simulink model "calc2"  (R2021a)
settings: Solver=VariableStepAuto  StartTime=0.0  StopTime=10.0  RelTol=1e-3
settings Model: Creator=Noha  LastModifiedBy=Noha

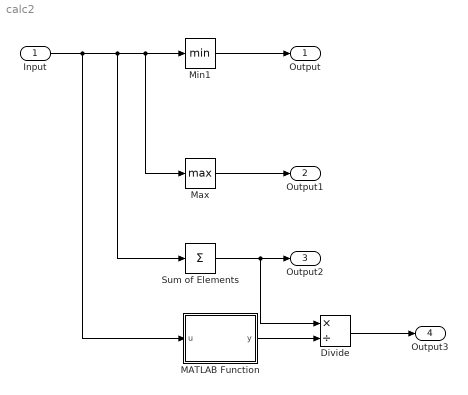
== system calc2 ==
  Input : Inport
  Divide : Product  Inputs=*/
  MATLAB Function : MATLAB Function  TreatAsAtomicUnit=on
  Max : MinMax  Function=max
  Min1 : MinMax
  Sum of Elements : Sum  Inputs=+
  Output : Outport
  Output1 : Outport  Port=2
  Output2 : Outport  Port=3
  Output3 : Outport  Port=4
  wires:
  Input/1 -> MATLAB Function/1(u), Sum of Elements/1, Max/1, Min1/1
  Min1/1 -> Output/1
  Max/1 -> Output1/1
  Sum of Elements/1 -> Output2/1, Divide/1
  MATLAB Function/1(y) -> Divide/2
  Divide/1 -> Output3/1

== matlab function calc2/MATLAB Function ==
  data: u input; y output
function y = fcn(u)

y = length(u);
